simulink model "FX150_model"  (R2022a)
settings: Solver=ode4  StartTime=0.0  StopTime=35  FixedStep=0.001  RelTol=1e-3
PreLoadFcn:
  | filepath  = fileparts(get_param(bdroot, 'FileName'))
  | cd(filepath);
InitFcn:
  | Model_Params;
values from neighbouring files (symbols this model uses):
  aM = 0.03    [Model_Params.m]
  aT = 1.4874    [Model_Params.m]
  bT = -0.0147    [Model_Params.m]
  ModelParam_envAltitude = -50    [Model_Params.m]
  ModelParam_GlobalNoiseGainSwitch = 0.4    [Model_Params.m]
  ModelParam_GPSEphFinal = 0.3    [Model_Params.m]
  ModelParam_GPSEpvFinal = 0.4    [Model_Params.m]
  ModelParam_GPSFix3DFix = 3    [Model_Params.m]
  ModelParam_GPSSatsVisible = 10    [Model_Params.m]
  ModelParam_motorJm = 0    [Model_Params.m]
  ModelParam_noiseBaroCoupleWithSpeed = 0    [Model_Params.m]
  ModelParam_noiseGPSSampTime = 0.2    [Model_Params.m]
  ModelParam_noisePowerIMU = 0    [Model_Params.m]
  ModelParam_noisePowerOffGainAccel = 0.04    [Model_Params.m]
  ModelParam_noisePowerOffGainAccelZ = 0.03    [Model_Params.m]
  ModelParam_noisePowerOffGainGyro = 0.02    [Model_Params.m]
  ModelParam_noisePowerOffGainGyroZ = 0.025    [Model_Params.m]
  ModelParam_noisePowerOffGainMag = 0.02    [Model_Params.m]
  ModelParam_noisePowerOffGainMagZ = 0.035    [Model_Params.m]
  ModelParam_noisePowerOnGainAccel = 0.8    [Model_Params.m]
  ModelParam_noisePowerOnGainAccelZ = 4.5    [Model_Params.m]
  ModelParam_noisePowerOnGainGyro = 2    [Model_Params.m]
  ModelParam_noisePowerOnGainGyroZ = 1    [Model_Params.m]
  ModelParam_noisePowerOnGainMag = 0.025    [Model_Params.m]
  ModelParam_noisePowerOnGainMagZ = 0.05    [Model_Params.m]
  ModelParam_noiseSampleTimeAccel = 0.001    [Model_Params.m]
  ModelParam_noiseSampleTimeGyro = 0.001    [Model_Params.m]
  ModelParam_noiseSampleTimeMag = 0.01    [Model_Params.m]
  ModelParam_noiseUpperGPS = 0.5    [Model_Params.m]
  ModelParam_noiseUpperWindBodyRatio = 0    [Model_Params.m]
  ModelParam_noiseWindSampTime = 0.001    [Model_Params.m]
  ModelParam_timeSampBaro = 0.01    [Model_Params.m]
  ModelParam_uavCCm = [0.0123 0.0123 0.0121]    [Model_Params.m]
  ModelParam_uavCd = [0.6023, 0.6023, 0.9]    [Model_Params.m]
  ModelParam_uavMass = 0.3175    [Model_Params.m]
  ModelParam_uavR = 0.075    [Model_Params.m]
  ModelParam_uavType = int8(3)    [Model_Params.m]
  w1 = 0.3812e+04    (= 3812)    [Model_Params.m]
  w2 = -1.3923e+04    (= -13923)    [Model_Params.m]
  w3 = 3.1012e+04    (= 31012)    [Model_Params.m]
undefined symbols (not defined in the file or in its folder): Earth, ModelParam_GPSEpvInitial, ModelParam_GPSEpvTimeConstant, ModelParam_noiseLowPassFilterCoeAccel, ModelParam_noiseLowPassFilterCoeGyro, ModelParam_timeSamp, Newton, Raphson, WGS84
libraries: simulink x4, aerolibtransform2 x3, sharedtransform x3, aerolibasang x3, aerolibatmos2 x2, aerolibutil x2, aerolibconvert2 x1, aerolibobsolete x1, shared6dof x1, aerolibnav x1, aerolibgravity2 x1
(part 1 of 2)
settings Model: SimulationMode=accelerator  Creator=Jinrui  LastModifiedBy=Lenovo
settings SolverCC: AlgebraicLoopSolver=TrustRegion
settings DataIOCC: ReturnWorkspaceOutputs=off
settings OptimizationCC: ZeroExternalMemoryAtStartup=off  ZeroInternalMemoryAtStartup=off  EfficientTunableParamExpr=on
settings DebuggingCC: ParameterTunabilityLossMsg=error  UnconnectedInputMsg=warning  UnconnectedOutputMsg=warning  UnconnectedLineMsg=warning  SFMachineParentedDataDiag=warning  ArithmeticOperatorsInVariantConditions=warning
settings SFSimCC: SimUseLocalCustomCode=off  MATLABDynamicMemAlloc=off  CustomCodeUndefinedFunction=UseInterfaceOnly  SimTargetLang=C++
settings RTWCC: SystemTargetFile=ert.tlc  GenerateMakefile=off  PackageGeneratedCodeAndArtifacts=on  PackageName=MulticopterModel  TemplateMakefile=ert_default_tmf  RTWUseLocalCustomCode=off  TargetLang=C++  RTWCompilerOptimization=on
settings CodeAppCC: ForceParamTrailComments=on  OperatorAnnotations=on  SimulinkDataObjDesc=on  SFDataObjDesc=on  MATLABFcnDesc=on  InsertBlockDesc=on  StateflowObjectComments=on  MATLABSourceComments=on
settings ERTTargetCC: TargetLangStandard=C++03 (ISO)  MultiwordLength=2048  GenerateSampleERTMain=on  CodeInterfacePackaging=C++ class  SupportContinuousTime=on  MultiInstanceErrorCode=None  RootIOFormat=Structure reference  ERTCustomFileTemplate=example_file_process.tlc  ERTFilePackagingFormat=Compact
settings SimscapeCC: SimscapeNormalizeSystem=off

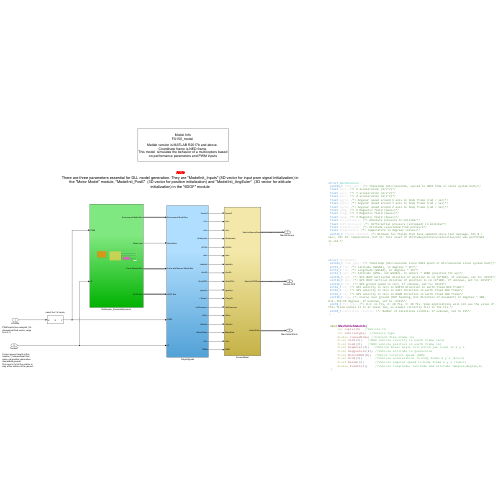
[thumbnail: Simulink's stored preview of the top-level diagram]
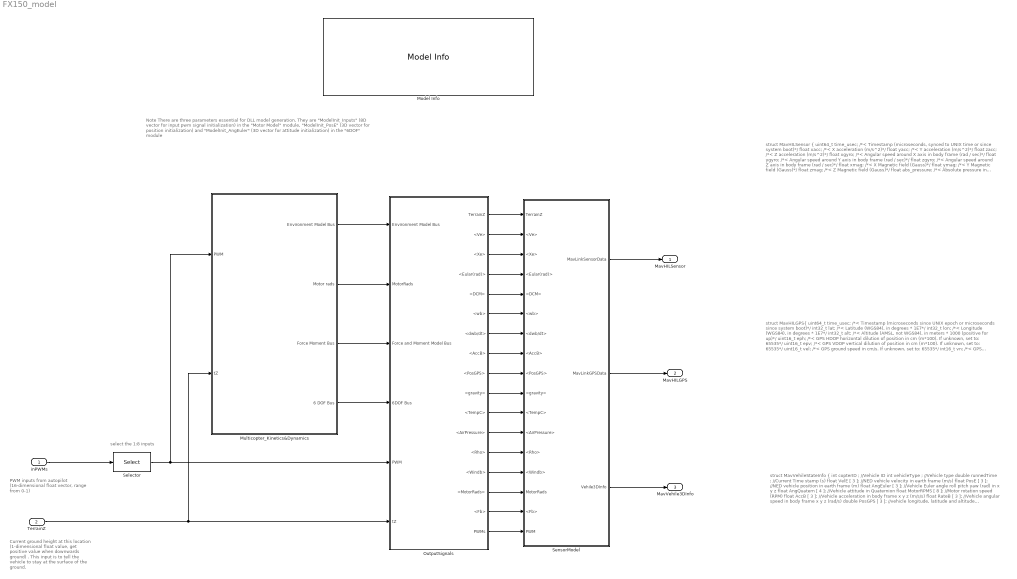
== system FX150_model ==
  note: PWM inputs from autopilot (16-dimensional float vector, range from 0-1)
  note: Note
      | There are three parameters essential for DLL model generation. They are "ModelInit_Inputs" (8D vector for input pwm signal initialization) in the "Motor Model" module, "ModelInit_PosE" (3D vector for position initialization) and "ModelInit_AngEuler" (3D vector for attitude initialization) in the "6DOF" module
  note: select the 1:8 inputs
  note: struct MavVehileStateInfo {
      | int copterID ; //Vehicle ID
      | int vehicleType ; //Vehicle type
      | double runnedTime ; //Current Time stamp (s)
      | float VelE [ 3 ]; //NED vehicle velocity in earth frame (m/s)
      | float PosE [ 3 ]; //NED vehicle position in earth frame (m)
      | float AngEuler [ 3 ]; //Vehicle Euler angle roll pitch yaw (rad) in x y z
      | float AngQuatern [ 4 ]; //Vehicle attitude in Quaternion
      | float MotorRPMS [ 8 ]; //Motor rotation speed (RPM)
      | float AccB [ 3 ]; //Vehicle acceleration in body frame x y z (m/s/s)
      | float RateB [ 3 ]; //Vehicle angular speed in body frame x y z (rad/s)
      | double PosGPS [ 3 ]; //vehicle longitude, latitude and altitude (degree,degree,m)
      | }
  note: struct MavHILGPS{
      | uint64_t time_usec; /*< Timestamp (microseconds since UNIX epoch or microseconds since system boot)*/
      | int32_t lat; /*< Latitude (WGS84), in degrees * 1E7*/
      | int32_t lon; /*< Longitude (WGS84), in degrees * 1E7*/
      | int32_t alt; /*< Altitude (AMSL, not WGS84), in meters * 1000 (positive for up)*/
      | uint16_t eph; /*< GPS HDOP horizontal dilution of position in cm (m*100). If unknown, set to: 65535*/
      | uint16_t epv; /*< GPS VDOP vertical dilution of position in cm (m*100). If unknown, set to: 65535*/
      | uint16_t vel; /*< GPS ground speed in cm/s. If unknown, set to: 65535*/
      | int16_t vn; /*< GPS velocity in cm/s in NORTH direction in earth-fixed NED frame*/
      | int16_t ve; /*< GPS velocity in cm/s in EAST direction in earth-fixed NED frame*/
      | int16_t vd; /*< GPS velocity in cm/s in DOWN direction in earth-fixed NED frame*/
      | uint16_t cog; /*< Course over ground (NOT heading, but direction of movement) in degrees * 100, 0.0..359.99 degrees. If unknown, set to: 65535*/
      | uint8_t fix_type; /*< 0-1: no fix, 2: 2D fix, 3: 3D fix. Some applications will not use the value of this field unless it is at least two, so always correctly fill in the fix.*/
      | uint8_t satellites_visible; /*< Number of satellites visible. If unknown, set to 255*/
      | }) ;
  note: struct MavHILSensor {
      | uint64_t time_usec; /*< Timestamp (microseconds, synced to UNIX time or since system boot)*/
      | float xacc; /*< X acceleration (m/s^2)*/
      | float yacc; /*< Y acceleration (m/s^2)*/
      | float zacc; /*< Z acceleration (m/s^2)*/
      | float xgyro; /*< Angular speed around X axis in body frame (rad / sec)*/
      | float ygyro; /*< Angular speed around Y axis in body frame (rad / sec)*/
      | float zgyro; /*< Angular speed around Z axis in body frame (rad / sec)*/
      | float xmag; /*< X Magnetic field (Gauss)*/
      | float ymag; /*< Y Magnetic field (Gauss)*/
      | float zmag; /*< Z Magnetic field (Gauss)*/
      | float abs_pressure; /*< Absolute pressure in millibar*/
      | float diff_pressure; /*< Differential pressure (airspeed) in millibar*/
      | float pressure_alt; /*< Altitude calculated from pressure*/
      | float temperature; /*< Temperature in degrees celsius*/
      | uint32_t fields_updated; /*< Bitmask for fields that have updated since last message, bit 0 = xacc, bit 12: temperature, bit 31: full reset of attitude/position/velocities/etc was performed in sim.*/
      | });
  note: Current ground height at this location (1-dimensional float value, get positive value when downwards ground) .
      | This input is to tell the vehicle to stay at the surface of the ground.
  inPWMs : Inport  PortDimensions=16
  TerrainZ : Inport  Port=2
  Model Info : simulink/Model-Wide Utilities/Model Info  Frame=on  DisplayStringWithTags=|  HorizontalTextAlignment=Center  LeftAlignmentValue=0.5
      | Model Info
      | %<ModelName> 
      | %<Description>   
      | Matlab version is MATLAB R2017b and above. 
      | Coordinate frame is NED frame.
      |  This model  simulates the behavior of a multicopters based 
      | on performance parameters and PWM inputs
  Multicopter_Kinetics&Dynamics : Subsystem
  OutputSignals : Subsystem
  Selector : Selector  InputPortWidth=16  IndexOptions=Index vector (dialog)  Indices=[1:8]  OutputSizes=1
  SensorModel : Subsystem
  MavHILSensor : Outport  OutDataTypeStr=Bus: MavLinkSensor  VectorParamsAs1DForOutWhenUnconnected=off
  MavHILGPS : Outport  Port=2  OutDataTypeStr=Bus: MavLinkGPS  VectorParamsAs1DForOutWhenUnconnected=off
  MavVehile3DInfo : Outport  Port=3  OutDataTypeStr=Bus: MavVehileInfo  VectorParamsAs1DForOutWhenUnconnected=off
  wires:
  inPWMs/1 -> Selector/1
  OutputSignals/9(<PosGPS>) -> SensorModel/9(<PosGPS>)
  SensorModel/2(MavLinkGPSData) -> MavHILGPS/1
  OutputSignals/1(TerrainZ) -> SensorModel/1(TerrainZ)
  OutputSignals/4(<Eular(rad)>) -> SensorModel/4(<Eular(rad)>)
  SensorModel/3(Vehile3DInfo) -> MavVehile3DInfo/1
  OutputSignals/2(<Ve>) -> SensorModel/2(<Ve>)
  OutputSignals/6(<wb>) -> SensorModel/6(<wb>)
  OutputSignals/5(<DCM>) -> SensorModel/5(<DCM>)
  SensorModel/1(MavLinkSensorData) -> MavHILSensor/1
  OutputSignals/15(<MotorRads>) -> SensorModel/15(MotorRads)
  OutputSignals/10(<gravity>) -> SensorModel/10(<gravity>)
  OutputSignals/7(<dwb/dt>) -> SensorModel/7(<dwb/dt>)
  OutputSignals/13(<Rho>) -> SensorModel/13(<Rho>)
  OutputSignals/3(<Xe>) -> SensorModel/3(<Xe>)
  OutputSignals/11(<TempC>) -> SensorModel/11(<TempC>)
  OutputSignals/12(<AirPressure>) -> SensorModel/12(<AirPressure>)
  OutputSignals/8(<AccB>) -> SensorModel/8(<AccB>)
  OutputSignals/16(<Fb>) -> SensorModel/16(<Fb>)
  OutputSignals/14(<Windb>) -> SensorModel/14(<Windb>)
  OutputSignals/17(PWMs) -> SensorModel/17(PWM)
  Selector/1 -> Multicopter_Kinetics&Dynamics/1(PWM), OutputSignals/5(PWM)
  Multicopter_Kinetics&Dynamics/1(Environment Model Bus) -> OutputSignals/1(Environment Model Bus)
  TerrainZ/1 -> Multicopter_Kinetics&Dynamics/2(tZ), OutputSignals/6(tZ)
  Multicopter_Kinetics&Dynamics/3(Force Moment Bus) -> OutputSignals/3(Force and Moment Model Bus)
  Multicopter_Kinetics&Dynamics/4(6 DOF Bus) -> OutputSignals/4(6DOF Bus)
  Multicopter_Kinetics&Dynamics/2(Motor rads) -> OutputSignals/2(MotorRads)

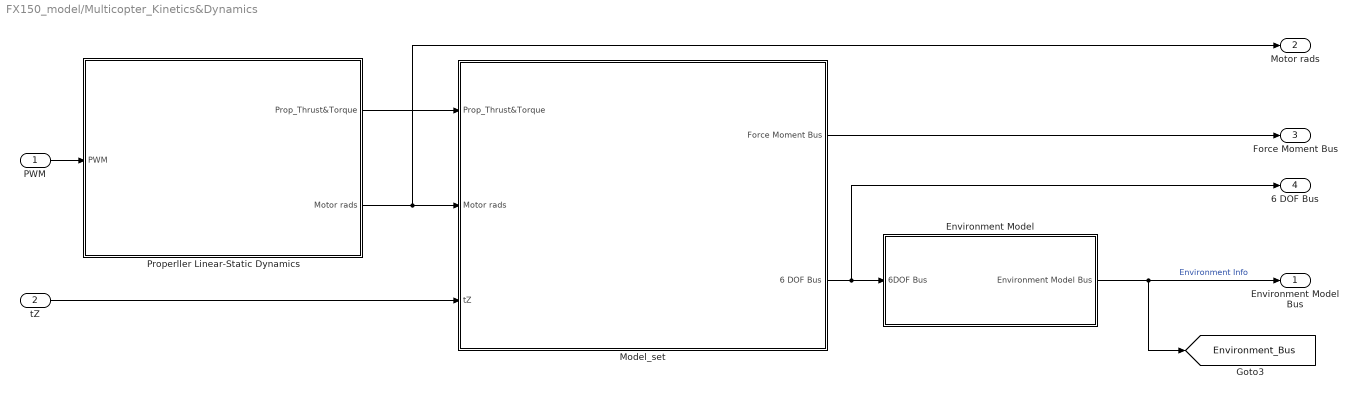
== system FX150_model/Multicopter_Kinetics&Dynamics ==
  PWM : Inport
  tZ : Inport  Port=2
  Environment Model : Subsystem
  Model_set : Subsystem
  Properller Linear-Static Dynamics : Subsystem  TreatAsAtomicUnit=on
  Environment Model Bus : Outport  VectorParamsAs1DForOutWhenUnconnected=off
  Motor rads : Outport  Port=2  VectorParamsAs1DForOutWhenUnconnected=off
  Force Moment Bus : Outport  Port=3  VectorParamsAs1DForOutWhenUnconnected=off
  6 DOF Bus : Outport  Port=4  VectorParamsAs1DForOutWhenUnconnected=off
  tag scope: Environment_Bus=global
  wires:
  Properller Linear-Static Dynamics/2(Motor rads) -> Motor rads/1, Model_set/2(Motor rads)
  tZ/1 -> Model_set/3(tZ)
  Model_set/2(6 DOF Bus) -> 6 DOF Bus/1, Environment Model/1(6DOF Bus)
  PWM/1 -> Properller Linear-Static Dynamics/1(PWM)
  Properller Linear-Static Dynamics/1(Prop_Thrust&Torque) -> Model_set/1(Prop_Thrust&Torque)
  Environment Model/1(Environment Model Bus) -> Environment Model Bus/1, [Environment_Bus]  "Environment Info"
  Model_set/1(Force Moment Bus) -> Force Moment Bus/1

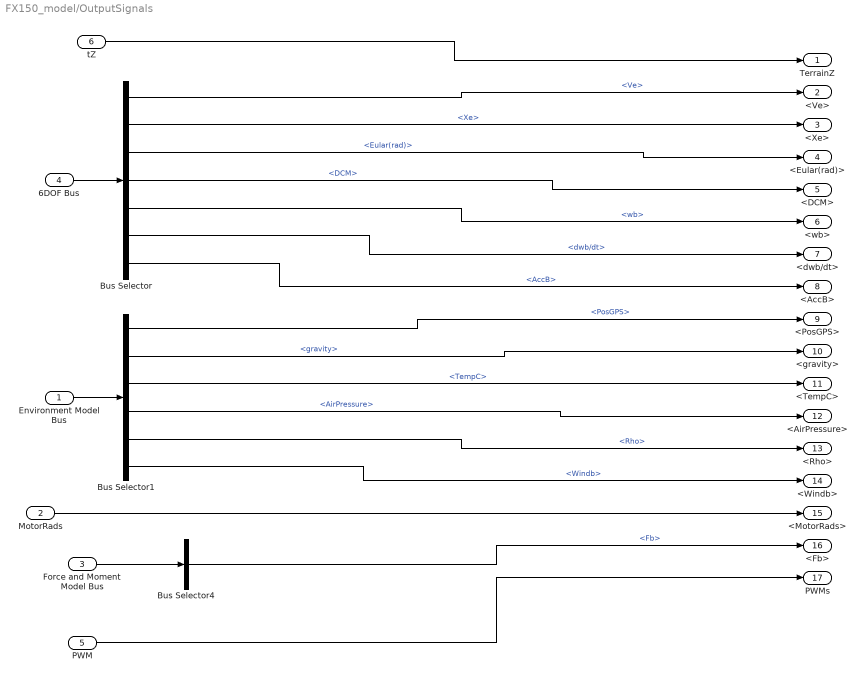
== system FX150_model/OutputSignals ==
  Environment Model Bus : Inport
  MotorRads : Inport  Port=2
  Force and Moment Model Bus : Inport  Port=3
  6DOF Bus : Inport  Port=4
  PWM : Inport  Port=5
  tZ : Inport  Port=6
  Bus Selector : BusSelector  OutputSignals=Ve,Xe,Eular(rad),DCM,wb,dwb/dt,AccB
  Bus Selector1 : BusSelector  OutputSignals=PosGPS,gravity,TempC,AirPressure,Rho,Windb
  Bus Selector4 : BusSelector  OutputSignals=Fb
  TerrainZ : Outport  VectorParamsAs1DForOutWhenUnconnected=off
  <Ve> : Outport  Port=2  VectorParamsAs1DForOutWhenUnconnected=off
  <Xe> : Outport  Port=3  VectorParamsAs1DForOutWhenUnconnected=off
  <Eular(rad)> : Outport  Port=4  VectorParamsAs1DForOutWhenUnconnected=off
  <DCM> : Outport  Port=5  VectorParamsAs1DForOutWhenUnconnected=off
  <wb> : Outport  Port=6  VectorParamsAs1DForOutWhenUnconnected=off
  <dwb/dt> : Outport  Port=7  VectorParamsAs1DForOutWhenUnconnected=off
  <AccB> : Outport  Port=8  VectorParamsAs1DForOutWhenUnconnected=off
  <PosGPS> : Outport  Port=9  VectorParamsAs1DForOutWhenUnconnected=off
  <gravity> : Outport  Port=10  VectorParamsAs1DForOutWhenUnconnected=off
  <TempC> : Outport  Port=11  VectorParamsAs1DForOutWhenUnconnected=off
  <AirPressure> : Outport  Port=12  VectorParamsAs1DForOutWhenUnconnected=off
  <Rho> : Outport  Port=13  VectorParamsAs1DForOutWhenUnconnected=off
  <Windb> : Outport  Port=14  VectorParamsAs1DForOutWhenUnconnected=off
  <MotorRads> : Outport  Port=15  VectorParamsAs1DForOutWhenUnconnected=off
  <Fb> : Outport  Port=16  VectorParamsAs1DForOutWhenUnconnected=off
  PWMs : Outport  Port=17  VectorParamsAs1DForOutWhenUnconnected=off
  wires:
  Force and Moment Model Bus/1 -> Bus Selector4/1
  MotorRads/1 -> <MotorRads>/1
  Bus Selector1/4 -> <AirPressure>/1  "<AirPressure>"
  Bus Selector/3 -> <Eular(rad)>/1  "<Eular(rad)>"
  Bus Selector1/6 -> <Windb>/1  "<Windb>"
  Bus Selector1/2 -> <gravity>/1  "<gravity>"
  PWM/1 -> PWMs/1
  Bus Selector/4 -> <DCM>/1  "<DCM>"
  Bus Selector/6 -> <dwb/dt>/1  "<dwb/dt>"
  Bus Selector1/1 -> <PosGPS>/1  "<PosGPS>"
  Bus Selector4/1 -> <Fb>/1  "<Fb>"
  Bus Selector/7 -> <AccB>/1  "<AccB>"
  Bus Selector/1 -> <Ve>/1  "<Ve>"
  Bus Selector/5 -> <wb>/1  "<wb>"
  Bus Selector/2 -> <Xe>/1  "<Xe>"
  Bus Selector1/5 -> <Rho>/1  "<Rho>"
  tZ/1 -> TerrainZ/1
  Bus Selector1/3 -> <TempC>/1  "<TempC>"
  Environment Model Bus/1 -> Bus Selector1/1
  6DOF Bus/1 -> Bus Selector/1

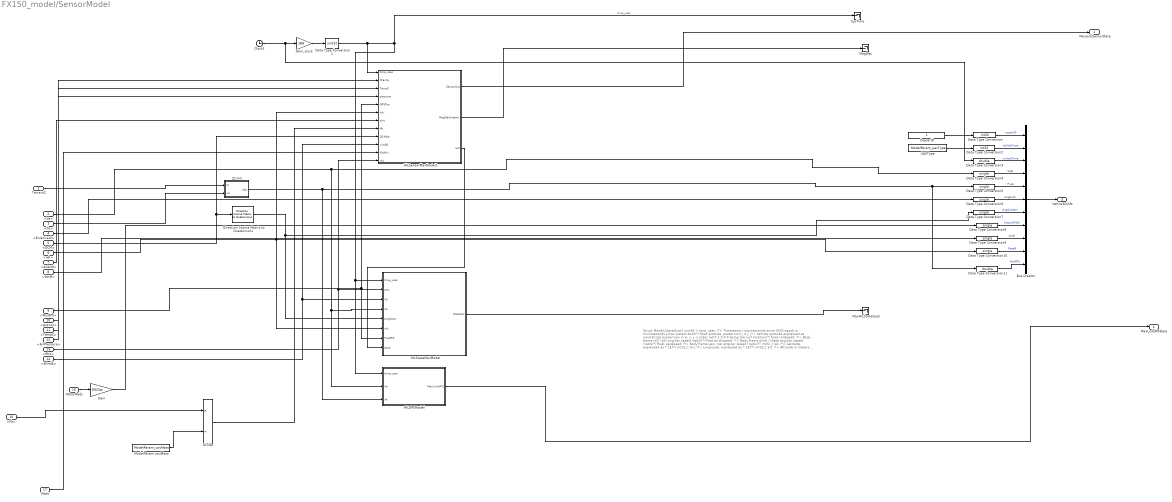
== system FX150_model/SensorModel ==
  note: Struct MavHILStateQuat{
      | uint64_t time_usec; /*< Timestamp (microseconds since UNIX epoch or microseconds since system boot)*/
      | float attitude_quaternion [ 4 ]; /*< Vehicle attitude expressed as normalized quaternion in w, x, y, z order (with 1 0 0 0 being the null-rotation)*/
      | float rollspeed; /*< Body frame roll / phi angular speed (rad/s)*/
      | float pitchspeed; /*< Body frame pitch / theta angular speed (rad/s)*/
      | float yawspeed; /*< Body frame yaw / psi angular speed (rad/s)*/
      | int32_t lat; /*< Latitude, expressed as * 1E7*/
      | int32_t lon; /*< Longitude, expressed as * 1E7*/
      | int32_t alt; /*< Altitude in meters, expressed as * 1000 (millimeters)*/
      | int16_t vx; /*< Ground X Speed (Latitude), expressed as cm/s*/
      | int16_t vy; /*< Ground Y Speed (Longitude), expressed as cm/s*/
      | int16_t vz; /*< Ground Z Speed (Altitude), expressed as cm/s*/
      | uint16_t ind_airspeed; /*< Indicated airspeed, expressed as cm/s*/
      | uint16_t true_airspeed; /*< True airspeed, expressed as cm/s*/
      | int16_t xacc; /*< X acceleration (mg)*/
      | int16_t yacc; /*< Y acceleration (mg)*/
      | int16_t zacc; /*< Z acceleration (mg)*/
      | };
  TerrainZ : Inport
  <Ve> : Inport  Port=2
  <Xe> : Inport  Port=3
  <Eular(rad)> : Inport  Port=4
  <DCM> : Inport  Port=5
  <wb> : Inport  Port=6
  <dwb/dt> : Inport  Port=7
  <AccB> : Inport  Port=8
  <PosGPS> : Inport  Port=9
  <gravity> : Inport  Port=10
  <TempC> : Inport  Port=11
  <AirPressure> : Inport  Port=12
  <Rho> : Inport  Port=13
  <Windb> : Inport  Port=14
  MotorRads : Inport  Port=15
  <Fb> : Inport  Port=16
  PWM : Inport  Port=17
  Bus Creator : BusCreator  Inputs=11  OutDataTypeStr=Bus: MavVehileInfo
  Clock1 : Clock
  CopterID : Constant
  Data Type Conversion : DataTypeConversion  OutDataTypeStr=int32  SaturateOnIntegerOverflow=off  RndMeth=Floor
  Data Type Conversion1 : DataTypeConversion  OutDataTypeStr=uint32  SaturateOnIntegerOverflow=off  RndMeth=Floor
  Data Type Conversion{4..10} (7 alike) : DataTypeConversion  OutDataTypeStr=single  SaturateOnIntegerOverflow=off  RndMeth=Floor
  Data Type Conversion11 : DataTypeConversion  OutDataTypeStr=double  SaturateOnIntegerOverflow=off  RndMeth=Floor
  Data Type Conversion2 : DataTypeConversion  OutDataTypeStr=int32  SaturateOnIntegerOverflow=off  RndMeth=Floor
  Data Type Conversion3 : DataTypeConversion  OutDataTypeStr=double  SaturateOnIntegerOverflow=off  RndMeth=Floor
  Direction Cosine Matrix to Quaternions : sharedtransform/Direction Cosine Matrix  to Quaternions  aMode=aMode  action=None  tolerance=eps(2)
      settings: SourceProductBaseCode=AE,PW,DR,MT,VE
  Divide : Product  Inputs=*/
  Gain : Gain  Gain=60/2/pi
  Gain_clock : Gain  Gain=1E6
  HILGPSModel : Subsystem
  HILSensorMavModel1 : Subsystem
  HILStateMavModel : Subsystem
  MagDec : Terminator
  MavHILStateQuat : Terminator
  ModelParam.uavMass : Constant  Value=ModelParam_uavMass
  SysTime : Terminator
  UAVType : Constant  Value=ModelParam_uavType
  ZLimit : MATLAB Function  TreatAsAtomicUnit=on
  MavLinkSensorData : Outport  VectorParamsAs1DForOutWhenUnconnected=off
  MavLinkGPSData : Outport  Port=2  VectorParamsAs1DForOutWhenUnconnected=off
  Vehile3DInfo : Outport  Port=3  VectorParamsAs1DForOutWhenUnconnected=off
  wires:
  <Xe>/1 -> ZLimit/2(xe)
  <PosGPS>/1 -> HILStateMavModel/7(PosGPS), HILSensorMavModel1/5(GPSPos)
  <TempC>/1 -> HILSensorMavModel1/3(TempC)
  <AirPressure>/1 -> HILSensorMavModel1/4(pressure)
  Clock1/1 -> Data Type Conversion3/1, Gain_clock/1
  Data Type Conversion1/1 -> HILSensorMavModel1/1(time_usec), SysTime/1, HILGPSModel/1(time_usec), HILStateMavModel/1(time_usec)  "time_usec"
  <gravity>/1 -> HILSensorMavModel1/2(Gravity)
  <Rho>/1 -> HILSensorMavModel1/12(rho), HILStateMavModel/2(pho)
  Gain_clock/1 -> Data Type Conversion1/1
  <DCM>/1 -> HILSensorMavModel1/9(DCMbe), Direction Cosine Matrix to Quaternions/1
  <Eular(rad)>/1 -> Data Type Conversion6/1
  <dwb/dt>/1 -> HILSensorMavModel1/7(dwt)
  <wb>/1 -> HILSensorMavModel1/6(wb), Data Type Conversion10/1, HILStateMavModel/6(wb)
  <Ve>/1 -> HILGPSModel/2(Ve), HILStateMavModel/4(Ve), Data Type Conversion4/1
  TerrainZ/1 -> ZLimit/1(zt)
  CopterID/1 -> Data Type Conversion/1
  HILSensorMavModel1/2(MagDeclination) -> MagDec/1
  <AccB>/1 -> Data Type Conversion9/1
  Divide/1 -> HILSensorMavModel1/8(Ab)
  Data Type Conversion5/1 -> Bus Creator/5  "PosE"
  Data Type Conversion7/1 -> Bus Creator/7  "AngQuatern"
  Data Type Conversion4/1 -> Bus Creator/4  "VelE"
  Data Type Conversion9/1 -> Bus Creator/9  "AccB"
  Data Type Conversion10/1 -> Bus Creator/10  "RateB"
  PWM/1 -> HILSensorMavModel1/11(PWMin)
  Data Type Conversion11/1 -> Bus Creator/11  "PosGPS"
  Data Type Conversion6/1 -> Bus Creator/6  "AngEuler"
  ZLimit/1(Xee) -> Data Type Conversion11/1, Data Type Conversion5/1, HILGPSModel/3(Xe)
  Data Type Conversion/1 -> Bus Creator/1  "copterID"
  Bus Creator/1 -> Vehile3DInfo/1
  <Fb>/1 -> Divide/1
  Gain/1 -> Data Type Conversion8/1
  HILStateMavModel/1(stateOut) -> MavHILStateQuat/1
  Data Type Conversion8/1 -> Bus Creator/8  "MotorRPMS"
  Direction Cosine Matrix to Quaternions/1 -> Data Type Conversion7/1, HILStateMavModel/5(AngQuat)
  UAVType/1 -> Data Type Conversion2/1
  Data Type Conversion3/1 -> Bus Creator/3  "runnedTime"
  HILSensorMavModel1/3(acc) -> HILStateMavModel/8(Accb)
  ModelParam.uavMass/1 -> Divide/2
  Data Type Conversion2/1 -> Bus Creator/2  "vehicleType"
  HILSensorMavModel1/1(SensorOut) -> MavLinkSensorData/1
  HILGPSModel/1(MavLinkGPS) -> MavLinkGPSData/1
  <Windb>/1 -> HILSensorMavModel1/10(windB), HILStateMavModel/3(Vb)
  MotorRads/1 -> Gain/1

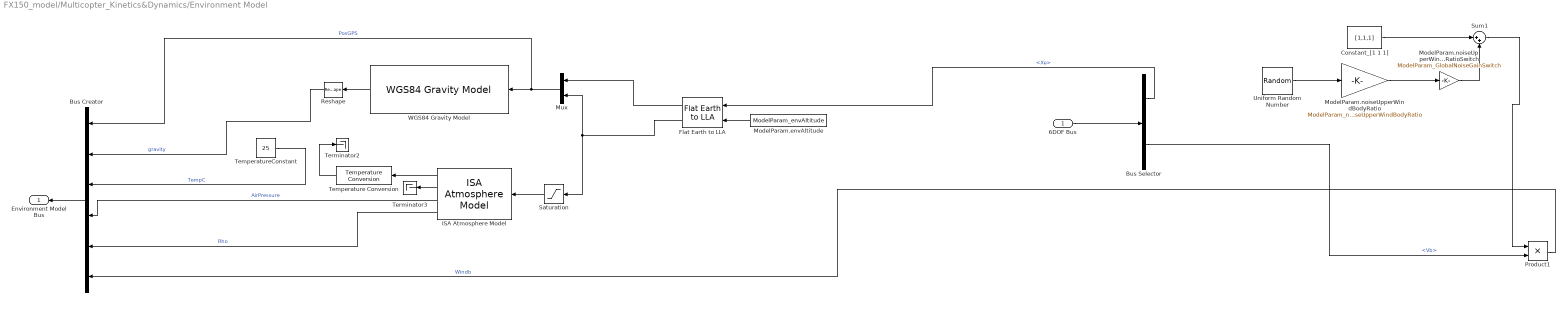
== system FX150_model/Multicopter_Kinetics&Dynamics/Environment Model ==
  6DOF Bus : Inport
  Bus Creator : BusCreator  Inputs=6
  Bus Selector : BusSelector  OutputSignals=Xe,Vb
  Constant_[1 1 1] : Constant  Value=[1,1,1]  VectorParams1D=off
  Flat Earth to LLA : aerolibtransform2/Flat Earth to LLA  units=Metric (MKS)  ptype=Earth (WGS84)  F=1/298.257223563  R=6378137  refPosPort=off  LL0=ModelParam_GPSLatLong  psi=0
  ISA Atmosphere Model : aerolibatmos2/ISA Atmosphere Model  custom=off  g=9.80665  gamma=1.4  R=287.0531  L=0.0065  h_trop=11000  h_strat=20000  rho0=1.225  P0=101325  T0=288.15  h0=0
  ModelParam.envAltitude : Constant  Value=ModelParam_envAltitude
  ModelParam.noiseUpperWindBodyRatio : Gain  Gain=ModelParam_noiseUpperWindBodyRatio
  ModelParam.noiseUpperWindBodyRatioSwitch : Gain  Gain=ModelParam_GlobalNoiseGainSwitch
  Mux : Mux  Inputs=2
  Product1 : Product
  Reshape : Reshape
  Saturation : Saturate  UpperLimit=100000  LowerLimit=0
  Sum1 : Sum  Inputs=|++
  Temperature Conversion : aerolibconvert2/Temperature Conversion  IU=K  OU=C
      settings: SourceProductBaseCode=AE
  TemperatureConstant : Constant  Value=25
  Terminator2 : Terminator
  Terminator3 : Terminator
  Uniform Random Number : UniformRandomNumber  Minimum=[-1,-1,-0.5]  Maximum=[1,1,0.5]  Seed=[564565,6846798,46545]  SampleTime=ModelParam_noiseWindSampTime
  "WGS84 Gravity Model " : aerolibobsolete/WGS84 Gravity Model   model=WGS84 Taylor Series  units=Metric (MKS)  no_atmos=on  precessing=on  jd_loc=off  month=October  day=10  year=2004  no_centrifugal=on  action=Warning
      settings: SourceProductBaseCode=AE
  Environment Model Bus : Outport  VectorParamsAs1DForOutWhenUnconnected=off
  wires:
  "WGS84 Gravity Model "/1 -> Reshape/1
  Reshape/1 -> Bus Creator/2  "gravity"
  ISA Atmosphere Model/1 -> Temperature Conversion/1
  ISA Atmosphere Model/2 -> Terminator3/1
  ISA Atmosphere Model/3 -> Bus Creator/4  "AirPressure"
  ISA Atmosphere Model/4 -> Bus Creator/5  "Rho"
  ModelParam.envAltitude/1 -> Flat Earth to LLA/2
  Mux/1 -> Bus Creator/1, "WGS84 Gravity Model "/1  "PosGPS"
  Flat Earth to LLA/1 -> Mux/1
  Bus Selector/2 -> Product1/2  "<Vb>"
  Uniform Random Number/1 -> ModelParam.noiseUpperWindBodyRatio/1
  Product1/1 -> Bus Creator/6  "Windb"
  Constant_[1 1 1]/1 -> Sum1/1
  ModelParam.noiseUpperWindBodyRatio/1 -> ModelParam.noiseUpperWindBodyRatioSwitch/1
  Sum1/1 -> Product1/1
  Temperature Conversion/1 -> Terminator2/1
  TemperatureConstant/1 -> Bus Creator/3  "TempC"
  ModelParam.noiseUpperWindBodyRatioSwitch/1 -> Sum1/2
  6DOF Bus/1 -> Bus Selector/1
  Bus Selector/1 -> Flat Earth to LLA/1  "<Xe>"
  Bus Creator/1 -> Environment Model Bus/1
  Flat Earth to LLA/2 -> Mux/2, Saturation/1
  Saturation/1 -> ISA Atmosphere Model/1

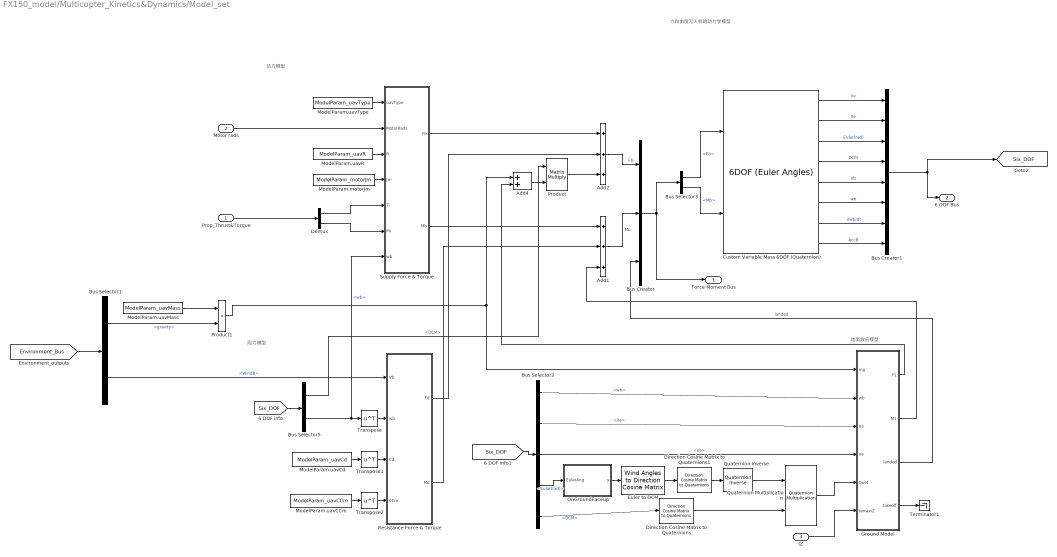
== system FX150_model/Multicopter_Kinetics&Dynamics/Model_set ==
  note: 地面效应模型
  note: 六自由度无人机的动力学模型
  note: 阻力模型
  note: 动力模型
  Prop_Thrust&Torque : Inport
  Motor rads : Inport  Port=2
  tZ : Inport  Port=3
  Add1 : Sum  Inputs=+++
  Add2 : Sum  Inputs=+++
  Add4 : Sum
  Bus Creator : BusCreator  Inputs=3
  Bus Creator1 : BusCreator  Inputs=8
  Bus Selector1 : BusSelector  OutputSignals=gravity,Windb
  Bus Selector2 : BusSelector  OutputSignals=wb,Xe,Ve,Eular(rad),DCM
  Bus Selector3 : BusSelector  OutputSignals=Fb,Mb
  Bus Selector5 : BusSelector  OutputSignals=DCM,wb
  Custom Variable Mass 6DOF (Quaternion) : shared6dof/6DOF (Euler Angles)  units=Metric (MKS)  mtype=Fixed  rep=Quaternion  xme_0=ModelInit_PosE  Vm_0=ModelInit_VelB  eul_0=ModelInit_AngEuler  pm_0=ModelInit_RateB  mass_0=ModelParam_uavMass  mass_e=0.5  mass_f=2.0  inertia=ModelParam_uavJ  inertia_e=eye(3)  inertia_f=2*eye(3)  k_quat=1.0  vre_flag=off  abi_flag=off  aMode=aMode  xme_statename=''  Vm_statename=''  eul_statename=''  quat_statename=''  pm_statename=''  mass_statename=''
      settings: SourceProductBaseCode=AE,PW,DR,MT,VE
  Demux : Demux  Outputs=2
  Direction Cosine Matrix to Quaternions : sharedtransform/Direction Cosine Matrix  to Quaternions  aMode=aMode  action=None  tolerance=eps(2)
      settings: SourceProductBaseCode=AE,PW,DR,MT,VE
  Direction Cosine Matrix to Quaternions1 : sharedtransform/Direction Cosine Matrix  to Quaternions  aMode=aMode  action=None  tolerance=eps(2)
      settings: SourceProductBaseCode=AE,PW,DR,MT,VE
  Euler to DCM : aerolibtransform2/Wind Angles to  Direction Cosine Matrix
      settings: SourceProductBaseCode=AE
  Ground Model : MATLAB Function  TreatAsAtomicUnit=on
  ModelParam.motorJm : Constant  Value=ModelParam_motorJm
  ModelParam.uavCCm : Constant  Value=ModelParam_uavCCm
  ModelParam.uavCd : Constant  Value=ModelParam_uavCd
  ModelParam.uavMass : Constant  Value=ModelParam_uavMass
  ModelParam.uavR : Constant  Value=ModelParam_uavR
  ModelParam.uavType : Constant  Value=ModelParam_uavType
  OnGroundFaceup : MATLAB Function  TreatAsAtomicUnit=on
  Product : Product  Multiplication=Matrix(*)
  Product1 : Product
  Quaternion Inverse : aerolibutil/Quaternion Inverse
  Quaternion Multiplication : aerolibutil/Quaternion Multiplication
  Resistance Force & Torque : MATLAB Function  TreatAsAtomicUnit=on
  Supply Force & Torque : MATLAB Function  TreatAsAtomicUnit=on
  Terminator1 : Terminator
  Transpose : Math  Operator=transpose  SignedPower=on
  Transpose1 : Math  Operator=transpose  SignedPower=on
  Transpose2 : Math  Operator=transpose  SignedPower=on
  Force Moment Bus : Outport  VectorParamsAs1DForOutWhenUnconnected=off
  6 DOF Bus : Outport  Port=2  VectorParamsAs1DForOutWhenUnconnected=off
  tag scope: Six_DOF=global
  wires:
  Bus Selector5/1 -> Product/1  "<DCM>"
  ModelParam.uavMass/1 -> Product1/1
  Transpose/1 -> Resistance Force & Torque/2(wb)
  Product1/1 -> Add4/1, Ground Model/1(mg)
  ModelParam.uavCd/1 -> Transpose1/1
  Supply Force & Torque/1(Fb) -> Add2/1
  Bus Selector2/4 -> OnGroundFaceup/1(EulerAng)  "<Eular(rad)>"
  Direction Cosine Matrix to Quaternions/1 -> Quaternion Multiplication/2
  ModelParam.uavR/1 -> Supply Force & Torque/3(R)
  Resistance Force & Torque/1(Fd) -> Add2/2
  Resistance Force & Torque/2(Md) -> Add1/2
  ModelParam.uavCCm/1 -> Transpose2/1
  Quaternion Inverse/1 -> Quaternion Multiplication/1
  ModelParam.motorJm/1 -> Supply Force & Torque/4(Jm)
  ModelParam.uavType/1 -> Supply Force & Torque/1(uavType)
  Bus Selector5/2 -> Supply Force & Torque/7(wb), Transpose/1  "<wb>"
  Demux/2 -> Supply Force & Torque/6(Mi)
  Transpose2/1 -> Resistance Force & Torque/4(CCm)
  Add1/1 -> Bus Creator/2  "Mb"
  Bus Selector2/3 -> Ground Model/4(Ve)  "<Ve>"
  Prop_Thrust&Torque/1 -> Demux/1
  [Six_DOF] -> Bus Selector5/1
  Product/1 -> Add2/3
  Demux/1 -> Supply Force & Torque/5(Ti)
  Bus Selector1/1 -> Product1/2  "<gravity>"
  Motor rads/1 -> Supply Force & Torque/2(MotorRads)
  Supply Force & Torque/2(Mb) -> Add1/1
  Bus Selector1/2 -> Resistance Force & Torque/1(Vb)  "<Windb>"
  Add2/1 -> Bus Creator/1  "Fb"
  [Six_DOF] -> Bus Selector2/1
  [Environment_Bus] -> Bus Selector1/1
  Transpose1/1 -> Resistance Force & Torque/3(Cd)
  Ground Model/4(takeoff) -> Terminator1/1
  Bus Selector2/5 -> Direction Cosine Matrix to Quaternions/1  "<DCM>"
  Quaternion Multiplication/1 -> Ground Model/5(Quet)
  tZ/1 -> Ground Model/6(terrainZ)
  Add4/1 -> Product/2
  Ground Model/3(landed) -> Bus Creator/3  "landed"
  Bus Selector2/1 -> Ground Model/2(wb)  "<wb>"
  Bus Selector2/2 -> Ground Model/3(Xe)  "<Xe>"
  Direction Cosine Matrix to Quaternions1/1 -> Quaternion Inverse/1
  OnGroundFaceup/1(y) -> Euler to DCM/1
  Euler to DCM/1 -> Direction Cosine Matrix to Quaternions1/1
  Ground Model/1(F1) -> Add4/2
  Ground Model/2(M1) -> Add1/3
  Bus Selector3/1 -> Custom Variable Mass 6DOF (Quaternion)/1  "<Fb>"
  Custom Variable Mass 6DOF (Quaternion)/7 -> Bus Creator1/7  "dwb/dt"
  Bus Creator/1 -> Bus Selector3/1, Force Moment Bus/1
  Custom Variable Mass 6DOF (Quaternion)/1 -> Bus Creator1/1  "Ve"
  Custom Variable Mass 6DOF (Quaternion)/2 -> Bus Creator1/2  "Xe"
  Bus Creator1/1 -> 6 DOF Bus/1, [Six_DOF]
  Custom Variable Mass 6DOF (Quaternion)/8 -> Bus Creator1/8  "AccB"
  Custom Variable Mass 6DOF (Quaternion)/6 -> Bus Creator1/6  "wb"
  Custom Variable Mass 6DOF (Quaternion)/5 -> Bus Creator1/5  "Vb"
  Bus Selector3/2 -> Custom Variable Mass 6DOF (Quaternion)/2  "<Mb>"
  Custom Variable Mass 6DOF (Quaternion)/4 -> Bus Creator1/4  "DCM"
  Custom Variable Mass 6DOF (Quaternion)/3 -> Bus Creator1/3  "Eular(rad)"

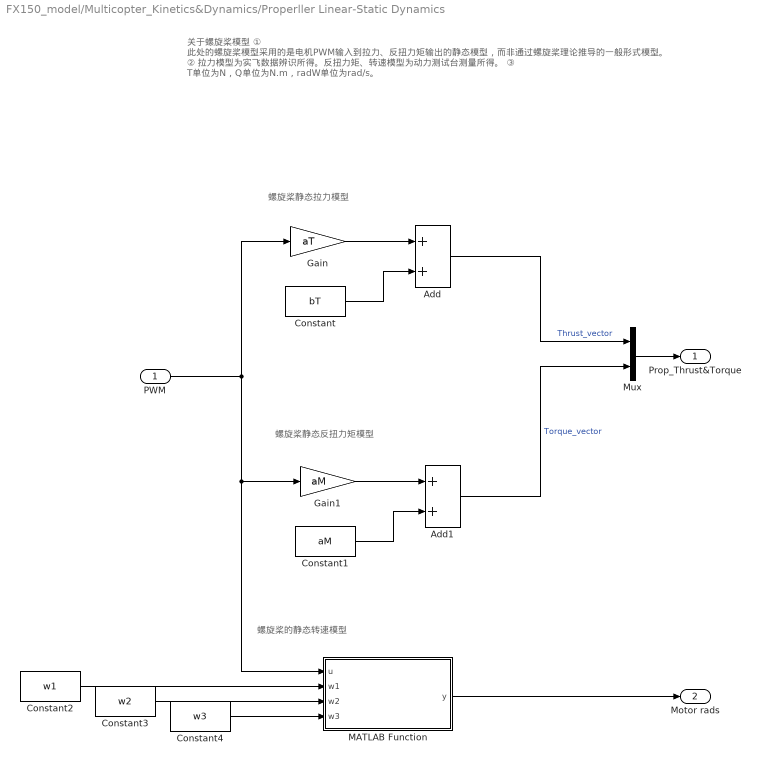
== system FX150_model/Multicopter_Kinetics&Dynamics/Properller Linear-Static Dynamics ==
  note: 螺旋桨的静态转速模型
  note: 关于螺旋桨模型
      | ① 此处的螺旋桨模型采用的是电机PWM输入到拉力、反扭力矩输出的静态模型，而非通过螺旋桨理论推导的一般形式模型。
      | ② 拉力模型为实飞数据辨识所得。反扭力矩、转速模型为动力测试台测量所得。
      | ③ T单位为N，Q单位为N.m，radW单位为rad/s。
  note: 螺旋桨静态反扭力矩模型
  note: 螺旋桨静态拉力模型
  PWM : Inport
  Add : Sum
  Add1 : Sum
  Constant : Constant  Value=bT
  Constant1 : Constant  Value=aM
  Constant2 : Constant  Value=w1
  Constant3 : Constant  Value=w2
  Constant4 : Constant  Value=w3
  Gain : Gain  Gain=aT
  Gain1 : Gain  Gain=aM
  MATLAB Function : MATLAB Function  TreatAsAtomicUnit=on
  Mux : Mux  Inputs=2
  Prop_Thrust&Torque : Outport  VectorParamsAs1DForOutWhenUnconnected=off
  Motor rads : Outport  Port=2  VectorParamsAs1DForOutWhenUnconnected=off
  wires:
  Gain/1 -> Add/1
  Constant/1 -> Add/2
  Add/1 -> Mux/1  "Thrust_vector"
  Add1/1 -> Mux/2  "Torque_vector"
  Constant1/1 -> Add1/2
  Gain1/1 -> Add1/1
  Mux/1 -> Prop_Thrust&Torque/1
  MATLAB Function/1(y) -> Motor rads/1
  PWM/1 -> Gain/1, MATLAB Function/1(u), Gain1/1
  Constant2/1 -> MATLAB Function/2(w1)
  Constant3/1 -> MATLAB Function/3(w2)
  Constant4/1 -> MATLAB Function/4(w3)

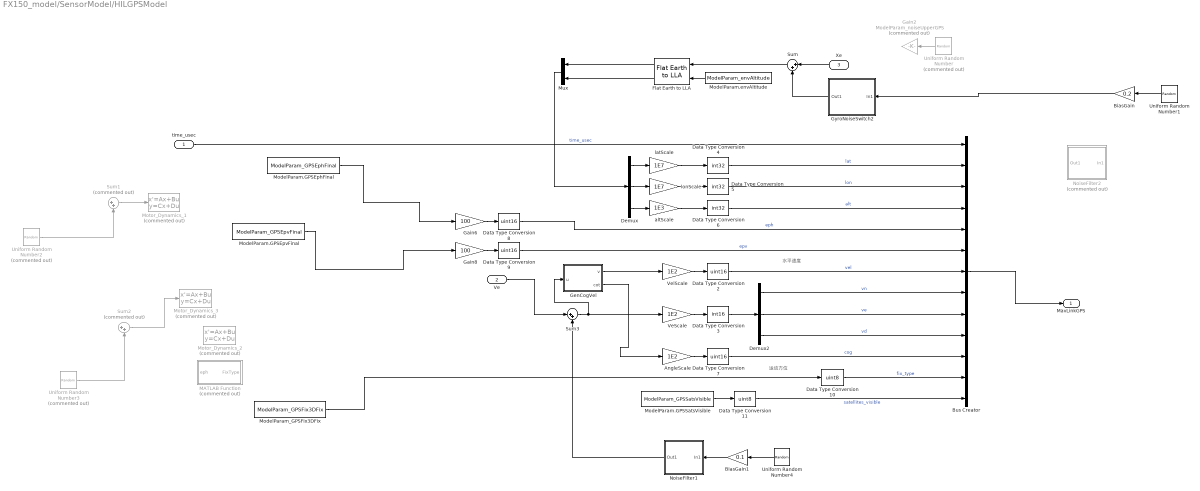
== system FX150_model/SensorModel/HILGPSModel ==
  note: 水平速度
  note: 运动方位
  time_usec : Inport
  Ve : Inport  Port=2
  Xe : Inport  Port=3
  AngleScale : Gain  Gain=1E2
  BiasGain : Gain  Gain=0.2
  BiasGain1 : Gain  Gain=0.1
  Bus Creator : BusCreator  Inputs=13  OutDataTypeStr=Bus: MavLinkGPS  NonVirtualBus=on
  Data Type Conversion10 : DataTypeConversion  OutDataTypeStr=uint8  RndMeth=Round  SaturateOnIntegerOverflow=off
  Data Type Conversion11 : DataTypeConversion  OutDataTypeStr=uint8  RndMeth=Round  SaturateOnIntegerOverflow=off
  Data Type Conversion{2,7..9} (4 alike) : DataTypeConversion  OutDataTypeStr=uint16  RndMeth=Round  SaturateOnIntegerOverflow=off
  Data Type Conversion3 : DataTypeConversion  OutDataTypeStr=int16  RndMeth=Round  SaturateOnIntegerOverflow=off
  Data Type Conversion4 : DataTypeConversion  OutDataTypeStr=int32  RndMeth=Round  SaturateOnIntegerOverflow=off
  Data Type Conversion5 : DataTypeConversion  OutDataTypeStr=int32  RndMeth=Round  SaturateOnIntegerOverflow=off
  Data Type Conversion6 : DataTypeConversion  OutDataTypeStr=int32  RndMeth=Round  SaturateOnIntegerOverflow=off
  Demux : Demux  Outputs=3
  Demux2 : Demux  Outputs=3
  Flat Earth to LLA : aerolibtransform2/Flat Earth to LLA  units=Metric (MKS)  ptype=Earth (WGS84)  F=1/298.257223563  R=6378137  refPosPort=off  LL0=ModelParam_GPSLatLong  psi=0
  Gain2 : Gain  Commented=on  Gain=ModelParam_noiseUpperGPS
  Gain6 : Gain  Gain=100
  Gain8 : Gain  Gain=100
  GenCogVel : MATLAB Function  TreatAsAtomicUnit=on
  GyroNoiseSwitch2 : Subsystem
  MATLAB Function : MATLAB Function  Commented=on  TreatAsAtomicUnit=on
  ModelParam.GPSEphFinal : Constant  Value=ModelParam_GPSEphFinal
  ModelParam.GPSEpvFinal : Constant  Value=ModelParam_GPSEpvFinal
  ModelParam.GPSSatsVisible : Constant  Value=ModelParam_GPSSatsVisible
  ModelParam.envAltitude : Constant  Value=ModelParam_envAltitude
  ModelParam_GPSFix3DFix : Constant  Value=ModelParam_GPSFix3DFix
  Motor_Dynamics_1 : StateSpace  Commented=on  A=-1/0.2  C=1/0.2  D=0  InitialCondition=20*0.2
  Motor_Dynamics_2 : StateSpace  Commented=on  A=-1/ModelParam_GPSEpvTimeConstant  C=1/ModelParam_GPSEpvTimeConstant  D=0  InitialCondition=ModelParam_GPSEpvInitial*ModelParam_GPSEpvTimeConstant
  Motor_Dynamics_3 : StateSpace  Commented=on  A=-1/0.2  C=1/0.2  D=0  InitialCondition=20*0.2
  Mux : Mux  Inputs=2
  NoiseFilter1 : Subsystem
  NoiseFilter2 : Subsystem  Commented=on
  Sum : Sum  Inputs=|++
  Sum1 : Sum  Commented=on  Inputs=|++
  Sum2 : Sum  Commented=on  Inputs=|++
  Sum3 : Sum  Inputs=|++
  Uniform Random Number : UniformRandomNumber  Commented=on  Minimum=[-1,-1,-3]  Maximum=[1,1,3]  Seed=[14524,7875,698]  SampleTime=ModelParam_timeSamp
  Uniform Random Number1 : UniformRandomNumber  Minimum=[-1,-1,-2]  Maximum=[1,1,2]  Seed=[1452,787,69]  SampleTime=ModelParam_noiseGPSSampTime
  Uniform Random Number2 : UniformRandomNumber  Commented=on  Minimum=-0.01  Maximum=0.01  Seed=4345454  SampleTime=ModelParam_noiseGPSSampTime
  Uniform Random Number3 : UniformRandomNumber  Commented=on  Seed=3244333  SampleTime=ModelParam_noiseGPSSampTime
  Uniform Random Number4 : UniformRandomNumber  Minimum=[-1,-1,-2]  Maximum=[1,1,2]  Seed=[5445,45433,33433]  SampleTime=ModelParam_noiseGPSSampTime
  VeScale : Gain  Gain=1E2
  VelScale : Gain  Gain=1E2
  altScale : Gain  Gain=1E3
  latScale : Gain  Gain=1E7
  lonScale : Gain  Gain=1E7
  MavLinkGPS : Outport  VectorParamsAs1DForOutWhenUnconnected=off
  wires:
  Data Type Conversion8/1 -> Bus Creator/5  "eph"
  Gain8/1 -> Data Type Conversion9/1
  Gain6/1 -> Data Type Conversion8/1
  Data Type Conversion9/1 -> Bus Creator/6  "epv"
  time_usec/1 -> Bus Creator/1  "time_usec"
  latScale/1 -> Data Type Conversion4/1
  lonScale/1 -> Data Type Conversion5/1
  altScale/1 -> Data Type Conversion6/1
  Data Type Conversion4/1 -> Bus Creator/2  "lat"
  Data Type Conversion5/1 -> Bus Creator/3  "lon"
  Data Type Conversion6/1 -> Bus Creator/4  "alt"
  Demux2/1 -> Bus Creator/8  "vn"
  Demux2/2 -> Bus Creator/9  "ve"
  Demux2/3 -> Bus Creator/10  "vd"
  VeScale/1 -> Data Type Conversion3/1
  Data Type Conversion3/1 -> Demux2/1
  VelScale/1 -> Data Type Conversion2/1
  Data Type Conversion2/1 -> Bus Creator/7  "vel"
  AngleScale/1 -> Data Type Conversion7/1
  Data Type Conversion7/1 -> Bus Creator/11  "cog"
  Data Type Conversion11/1 -> Bus Creator/13  "satellites_visible"
  Data Type Conversion10/1 -> Bus Creator/12  "fix_type"
  ModelParam.GPSSatsVisible/1 -> Data Type Conversion11/1
  Flat Earth to LLA/2 -> Mux/2
  ModelParam.envAltitude/1 -> Flat Earth to LLA/2
  Xe/1 -> Sum/1
  Flat Earth to LLA/1 -> Mux/1
  Demux/1 -> latScale/1
  Demux/2 -> lonScale/1
  Demux/3 -> altScale/1
  Uniform Random Number/1 -> Gain2/1
  Sum/1 -> Flat Earth to LLA/1
  Uniform Random Number1/1 -> BiasGain/1
  BiasGain/1 -> GyroNoiseSwitch2/1(In1)
  Mux/1 -> Demux/1
  ModelParam.GPSEphFinal/1 -> Gain6/1
  Sum2/1 -> Motor_Dynamics_3/1
  ModelParam_GPSFix3DFix/1 -> Data Type Conversion10/1
  Ve/1 -> Sum3/1
  GenCogVel/1(v) -> VelScale/1
  GyroNoiseSwitch2/1(Out1) -> Sum/2
  Bus Creator/1 -> MavLinkGPS/1
  BiasGain1/1 -> NoiseFilter1/1(In1)
  Uniform Random Number4/1 -> BiasGain1/1
  GenCogVel/2(cot) -> AngleScale/1
  Sum1/1 -> Motor_Dynamics_1/1
  Uniform Random Number2/1 -> Sum1/2
  Uniform Random Number3/1 -> Sum2/2
  ModelParam.GPSEpvFinal/1 -> Gain8/1
  Sum3/1 -> GenCogVel/1(u), VeScale/1
  NoiseFilter1/1(Out1) -> Sum3/2

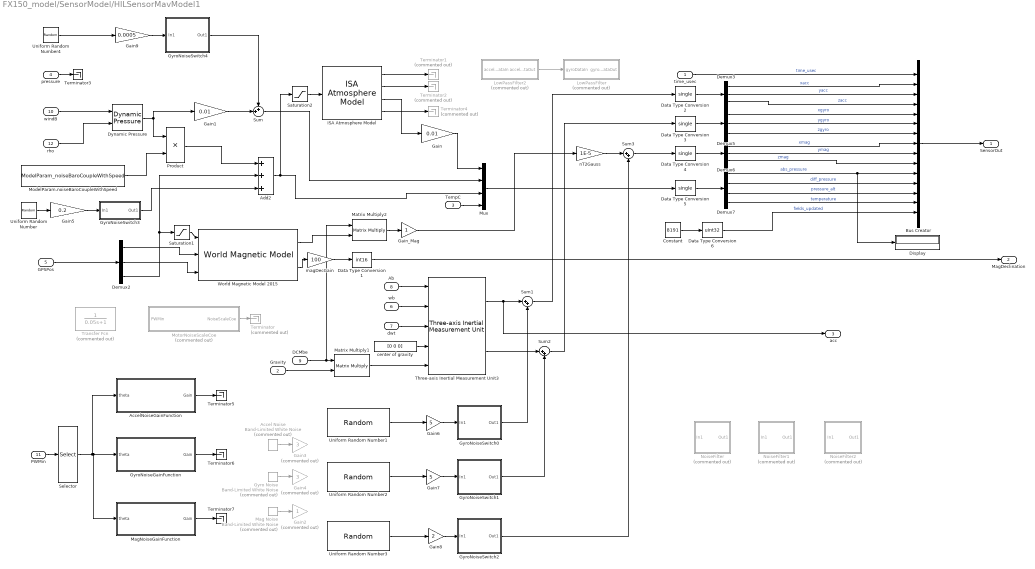
== system FX150_model/SensorModel/HILSensorMavModel1 ==
  time_usec : Inport
  Gravity : Inport  Port=2
  TempC : Inport  Port=3
  pressure : Inport  Port=4
  GPSPos : Inport  Port=5
  wb : Inport  Port=6
  dwt : Inport  Port=7
  Ab : Inport  Port=8
  DCMbe : Inport  Port=9
  windB : Inport  Port=10
  PWMin : Inport  Port=11
  rho : Inport  Port=12
  Accel Noise : simulink/Sources/Band-Limited White Noise  Commented=on  Cov=ModelParam_noisePowerAccel  Ts=ModelParam_noiseSampleTimeAccel  seed=[411144,1416,71144]
  AccelNoiseGainFunction : MATLAB Function  TreatAsAtomicUnit=on
  Add2 : Sum  Inputs=+++
  Bus Creator : BusCreator  Inputs=15  OutDataTypeStr=Bus: MavLinkSensor  NonVirtualBus=on
  Constant : Constant  Value=8191
  Data Type Conversion1 : DataTypeConversion  OutDataTypeStr=int16  SaturateOnIntegerOverflow=off  RndMeth=Floor
  Data Type Conversion{2..5} (4 alike) : DataTypeConversion  OutDataTypeStr=single  SaturateOnIntegerOverflow=off  RndMeth=Floor
  Data Type Conversion6 : DataTypeConversion  OutDataTypeStr=uint32  SaturateOnIntegerOverflow=off  RndMeth=Floor
  Demux{2..3,5..6} (4 alike) : Demux  Outputs=3
  Demux7 : Demux
  Display : Display
  Dynamic Pressure : aerolibasang/Dynamic Pressure
  Gain : Gain  Gain=0.01
  Gain1 : Gain  Gain=0.01
  Gain2 : Gain  Commented=on
  Gain3 : Gain  Commented=on  Gain=3
  Gain4 : Gain  Commented=on  Gain=3
  Gain5 : Gain  Gain=0.2
  Gain6 : Gain  Gain=5
  Gain7 : Gain  Gain=5
  Gain8 : Gain  Gain=2
  Gain9 : Gain  Gain=0.0005
  Gain_Mag : Gain
  Gyro Noise : simulink/Sources/Band-Limited White Noise  Commented=on  Cov=ModelParam_noisePowerGyro  Ts=ModelParam_noiseSampleTimeGyro  seed=[111,116,144]
  GyroNoiseGainFunction : MATLAB Function  TreatAsAtomicUnit=on
  GyroNoiseSwitch0 : Subsystem
  GyroNoiseSwitch1 : Subsystem
  GyroNoiseSwitch2 : Subsystem
  GyroNoiseSwitch3 : Subsystem
  GyroNoiseSwitch4 : Subsystem
  ISA Atmosphere Model : aerolibatmos2/ISA Atmosphere Model  custom=off  g=9.80665  gamma=1.4  R=287.0531  L=0.0065  h_trop=11000  h_strat=20000  rho0=1.225  P0=101325  T0=288.15  h0=0
  LowPassFilter : Subsystem  Commented=on
  LowPassFilter2 : Subsystem  Commented=on
  Mag Noise : simulink/Sources/Band-Limited White Noise  Commented=on  Cov=ModelParam_noisePowerMag  Ts=ModelParam_noiseSampleTimeMag  seed=[114,11699,999144]
  MagNoiseGainFunction : MATLAB Function  TreatAsAtomicUnit=on
  Matrix Multiply1 : Product  Multiplication=Matrix(*)
  Matrix Multiply2 : Product  Multiplication=Matrix(*)
  ModelParam.noiseBaroCoupleWithSpeed : Constant  Value=ModelParam_noiseBaroCoupleWithSpeed
  MotorNoiseScaleCoe : MATLAB Function  Commented=on  TreatAsAtomicUnit=on
  Mux : Mux
  NoiseFilter : Subsystem  Commented=on
  NoiseFilter1 : Subsystem  Commented=on
  NoiseFilter2 : Subsystem  Commented=on
  Product : Product
  Saturation1 : Saturate  UpperLimit=100000  LowerLimit=0
  Saturation2 : Saturate  UpperLimit=100000  LowerLimit=0
  Selector : Selector  InputPortWidth=8  IndexOptions=Index vector (dialog)  Indices=[1]  OutputSizes=1
  Sum : Sum  Inputs=++|
  Sum1 : Sum  Inputs=|++
  Sum2 : Sum  Inputs=|++
  Sum3 : Sum  Inputs=|++
  Terminator{,1..2,4} (4 alike) : Terminator  Commented=on
  Terminator{3,5..7} (4 alike) : Terminator
  Three-axis Inertial Measurement Unit3 : aerolibnav/Three-axis Inertial Measurement Unit  units=Metric (MKS)  imu=[0 0 0]  i_Ts=0  dtype_a=on  w_a=190  z_a=0.707  a_sf_cc=[1 0 0; 0 1 0; 0 0 1]  a_bias=[0 0 0]  a_sat="[-160  -160  -160 160 160 160]"  dtype_g=on  w_g=190  z_g=0.707  g_sf_cc=[1 0 0; 0 1 0; 0 0 1]  g_bias=[0 0 0]  g_sens=[0 0 0]  g_sat="[-4.36  -4.36  -4.36 4.36 4.36 4.36]"  i_rand=off  i_seeds=[23093 23094 23095 23096 23097 23098]  i_pow=ModelParam_noisePowerIMU*[0.0000005 0.0000005 0.0000005 0.000000002 0.000000002 0.000000002]
  Transfer Fcn : TransferFcn  Commented=on  Denominator=[0.05 1]
  Uniform Random Number : UniformRandomNumber  Minimum=-2  Maximum=2  Seed=15634  SampleTime=ModelParam_timeSampBaro
  Uniform Random Number1 : UniformRandomNumber  Minimum=-[0.1,0.1,0.2]  Maximum=[0.1,0.1,0.2]  Seed=[12233,645554,678766]  SampleTime=0.004
  Uniform Random Number2 : UniformRandomNumber  Minimum=-[0.01,0.01,0.01]  Maximum=[0.01,0.01,0.01]  Seed=[3243,44556,2334343]  SampleTime=0.004
  Uniform Random Number3 : UniformRandomNumber  Minimum=-[0.01,0.01,0.01]  Maximum=[0.01,0.01,0.01]  Seed=[45465,454534,1234232]  SampleTime=0.004
  Uniform Random Number4 : UniformRandomNumber  Seed=25634  SampleTime=0.01
  World Magnetic Model 2015 : aerolibgravity2/World Magnetic Model  model=WMM2015 V2 (2015-2020)  customFile='WMM2020.COF'  units=Metric (MKS)  time_in=off  month=November  day=3  year=2017  action=Error  h_out=off  dec_out=on  inc_out=off  ti_out=off
      settings: SourceProductBaseCode=AE
  center of gravity : Constant  Value=[0 0 0]
  magDecGain : Gain  Gain=100
  nT2Gauss : Gain  Gain=1E-5
  SensorOut : Outport  VectorParamsAs1DForOutWhenUnconnected=off
  MagDeclination : Outport  Port=2  VectorParamsAs1DForOutWhenUnconnected=off
  acc : Outport  Port=3  VectorParamsAs1DForOutWhenUnconnected=off
  wires:
  center of gravity/1 -> Three-axis Inertial Measurement Unit3/4
  Sum1/1 -> Data Type Conversion2/1
  Sum2/1 -> Data Type Conversion3/1
  Sum3/1 -> Data Type Conversion4/1
  Matrix Multiply2/1 -> Gain_Mag/1
  magDecGain/1 -> Data Type Conversion1/1
  GyroNoiseSwitch3/1(Out1) -> Add2/3
  Product/1 -> Add2/1
  ModelParam.noiseBaroCoupleWithSpeed/1 -> Product/2
  rho/1 -> Dynamic Pressure/2
  windB/1 -> Dynamic Pressure/1
  Uniform Random Number/1 -> Gain5/1
  dwt/1 -> Three-axis Inertial Measurement Unit3/3
  Gain_Mag/1 -> nT2Gauss/1
  Dynamic Pressure/1 -> Gain1/1, Product/1
  pressure/1 -> Terminator3/1
  Add2/1 -> Mux/3, Saturation2/1
  Demux2/3 -> Saturation1/1, Add2/2
  Demux2/2 -> World Magnetic Model 2015/3
  Demux2/1 -> World Magnetic Model 2015/2
  Matrix Multiply1/1 -> Three-axis Inertial Measurement Unit3/5
  DCMbe/1 -> Matrix Multiply2/1, Matrix Multiply1/1
  Gravity/1 -> Matrix Multiply1/2
  Sum/1 -> Mux/2
  Gain/1 -> Mux/1
  Data Type Conversion6/1 -> Bus Creator/15  "fields_updated"
  Constant/1 -> Data Type Conversion6/1
  time_usec/1 -> Bus Creator/1  "time_usec"
  GPSPos/1 -> Demux2/1
  Demux7/2 -> Bus Creator/12  "diff_pressure"
  Demux7/3 -> Bus Creator/13  "pressure_alt"
  Demux6/2 -> Bus Creator/9  "ymag"
  Demux6/3 -> Bus Creator/10  "zmag"
  TempC/1 -> Mux/4
  Mux/1 -> Data Type Conversion5/1
  Demux7/1 -> Bus Creator/11, Display/1  "abs_pressure"
  Demux5/2 -> Bus Creator/6  "ygyro"
  Demux6/1 -> Bus Creator/8  "xmag"
  Demux5/3 -> Bus Creator/7  "zgyro"
  Demux7/4 -> Bus Creator/14  "temperature"
  Demux3/1 -> Bus Creator/2  "xacc"
  Demux3/2 -> Bus Creator/3  "yacc"
  Demux5/1 -> Bus Creator/5  "xgyro"
  Demux3/3 -> Bus Creator/4  "zacc"
  PWMin/1 -> Selector/1
  Ab/1 -> Three-axis Inertial Measurement Unit3/1
  wb/1 -> Three-axis Inertial Measurement Unit3/2
  MotorNoiseScaleCoe/1(NoiseScaleCoe) -> Terminator/1
  Selector/1 -> AccelNoiseGainFunction/1(theta), MagNoiseGainFunction/1(theta), GyroNoiseGainFunction/1(theta)
  AccelNoiseGainFunction/1(Gain) -> Terminator5/1
  Mag Noise/1 -> Gain2/1
  nT2Gauss/1 -> Sum3/1
  Gain8/1 -> GyroNoiseSwitch2/1(In1)
  GyroNoiseSwitch1/1(Out1) -> Sum2/2
  GyroNoiseSwitch2/1(Out1) -> Sum3/2
  Data Type Conversion2/1 -> Demux3/1
  Data Type Conversion3/1 -> Demux5/1
  Data Type Conversion4/1 -> Demux6/1
  Data Type Conversion5/1 -> Demux7/1
  Bus Creator/1 -> SensorOut/1
  Data Type Conversion1/1 -> MagDeclination/1
  Three-axis Inertial Measurement Unit3/1 -> acc/1, Sum1/1
  Three-axis Inertial Measurement Unit3/2 -> Sum2/1
  ISA Atmosphere Model/2 -> Terminator2/1
  ISA Atmosphere Model/4 -> Terminator4/1
  ISA Atmosphere Model/1 -> Terminator1/1
  Gain5/1 -> GyroNoiseSwitch3/1(In1)
  Accel Noise/1 -> Gain3/1
  GyroNoiseSwitch0/1(Out1) -> Sum1/2
  Gyro Noise/1 -> Gain4/1
  GyroNoiseGainFunction/1(Gain) -> Terminator6/1
  MagNoiseGainFunction/1(Gain) -> Terminator7/1
  Uniform Random Number1/1 -> Gain6/1
  Gain7/1 -> GyroNoiseSwitch1/1(In1)
  Uniform Random Number2/1 -> Gain7/1
  Uniform Random Number3/1 -> Gain8/1
  ISA Atmosphere Model/3 -> Gain/1
  Gain6/1 -> GyroNoiseSwitch0/1(In1)
  LowPassFilter2/1(accelDataOut) -> LowPassFilter/1(gyroDataIn)
  Gain9/1 -> GyroNoiseSwitch4/1(In1)
  Uniform Random Number4/1 -> Gain9/1
  Gain1/1 -> Sum/2
  GyroNoiseSwitch4/1(Out1) -> Sum/1
  Saturation1/1 -> World Magnetic Model 2015/1
  Saturation2/1 -> ISA Atmosphere Model/1
  World Magnetic Model 2015/1 -> Matrix Multiply2/2
  World Magnetic Model 2015/2 -> magDecGain/1

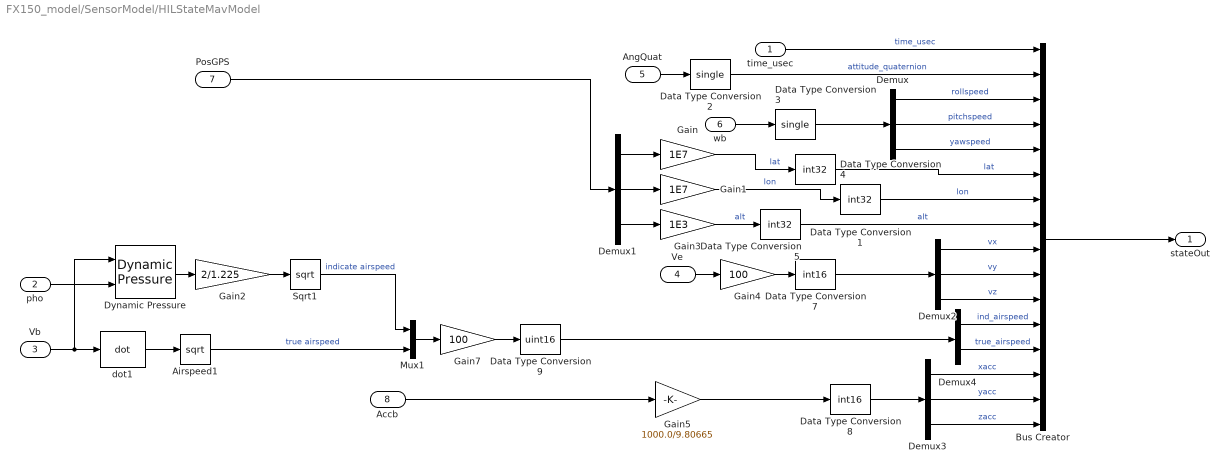
== system FX150_model/SensorModel/HILStateMavModel ==
  time_usec : Inport
  pho : Inport  Port=2
  Vb : Inport  Port=3
  Ve : Inport  Port=4
  AngQuat : Inport  Port=5
  wb : Inport  Port=6
  PosGPS : Inport  Port=7
  Accb : Inport  Port=8
  Airspeed1 : Sqrt  AlgorithmType=Newton-Raphson
  Bus Creator : BusCreator  Inputs=16  OutDataTypeStr=Bus: MavLinkStateQuat  NonVirtualBus=on
  Data Type Conversion1 : DataTypeConversion  OutDataTypeStr=int32  RndMeth=Round  SaturateOnIntegerOverflow=off
  Data Type Conversion2 : DataTypeConversion  OutDataTypeStr=single  SaturateOnIntegerOverflow=off  RndMeth=Floor
  Data Type Conversion3 : DataTypeConversion  OutDataTypeStr=single  SaturateOnIntegerOverflow=off  RndMeth=Floor
  Data Type Conversion4 : DataTypeConversion  OutDataTypeStr=int32  RndMeth=Round  SaturateOnIntegerOverflow=off
  Data Type Conversion5 : DataTypeConversion  OutDataTypeStr=int32  RndMeth=Round  SaturateOnIntegerOverflow=off
  Data Type Conversion7 : DataTypeConversion  OutDataTypeStr=int16  RndMeth=Round  SaturateOnIntegerOverflow=off
  Data Type Conversion8 : DataTypeConversion  OutDataTypeStr=int16  RndMeth=Round  SaturateOnIntegerOverflow=off
  Data Type Conversion9 : DataTypeConversion  OutDataTypeStr=uint16  RndMeth=Round  SaturateOnIntegerOverflow=off
  Demux{,1..3} (4 alike) : Demux  Outputs=3
  Demux4 : Demux  Outputs=2
  Dynamic Pressure : aerolibasang/Dynamic Pressure
  Gain : Gain  Gain=1E7
  Gain1 : Gain  Gain=1E7
  Gain2 : Gain  Gain=2/1.225
  Gain3 : Gain  Gain=1E3
  Gain4 : Gain  Gain=100
  Gain5 : Gain  Gain=1000.0/9.80665
  Gain7 : Gain  Gain=100
  Mux1 : Mux  Inputs=2
  Sqrt1 : Sqrt
  dot1 : aerolibasang/Incidence, Sideslip, & Airspeed/dot  SystemSampleTime=-1  VariantActivationTime=update diagram  Latency=0  AutoFrameSizeCalculation=off
      settings: SourceProductBaseCode=AE
  stateOut : Outport  VectorParamsAs1DForOutWhenUnconnected=off
  wires:
  Sqrt1/1 -> Mux1/1  "indicate airspeed"
  Gain2/1 -> Sqrt1/1
  Dynamic Pressure/1 -> Gain2/1
  time_usec/1 -> Bus Creator/1  "time_usec"
  Vb/1 -> dot1/1, Dynamic Pressure/1
  AngQuat/1 -> Data Type Conversion2/1
  Ve/1 -> Gain4/1
  wb/1 -> Data Type Conversion3/1
  Airspeed1/1 -> Mux1/2  "true airspeed"
  Mux1/1 -> Gain7/1
  Demux4/1 -> Bus Creator/12  "ind_airspeed"
  Demux4/2 -> Bus Creator/13  "true_airspeed"
  Demux3/3 -> Bus Creator/16  "zacc"
  Demux3/2 -> Bus Creator/15  "yacc"
  Demux3/1 -> Bus Creator/14  "xacc"
  Gain5/1 -> Data Type Conversion8/1
  Accb/1 -> Gain5/1
  Demux2/3 -> Bus Creator/11  "vz"
  Demux2/2 -> Bus Creator/10  "vy"
  Demux2/1 -> Bus Creator/9  "vx"
  Gain4/1 -> Data Type Conversion7/1
  Gain3/1 -> Data Type Conversion5/1  "alt"
  Gain1/1 -> Data Type Conversion1/1  "lon"
  Gain/1 -> Data Type Conversion4/1  "lat"
  Demux1/3 -> Gain3/1
  Demux1/2 -> Gain1/1
  Demux1/1 -> Gain/1
  Demux/3 -> Bus Creator/5  "yawspeed"
  Demux/2 -> Bus Creator/4  "pitchspeed"
  Demux/1 -> Bus Creator/3  "rollspeed"
  Data Type Conversion2/1 -> Bus Creator/2  "attitude_quaternion"
  pho/1 -> Dynamic Pressure/2
  Gain7/1 -> Data Type Conversion9/1
  dot1/1 -> Airspeed1/1
  Data Type Conversion3/1 -> Demux/1
  Data Type Conversion7/1 -> Demux2/1
  Data Type Conversion9/1 -> Demux4/1
  Data Type Conversion8/1 -> Demux3/1
  Data Type Conversion4/1 -> Bus Creator/6  "lat"
  Data Type Conversion1/1 -> Bus Creator/7  "lon"
  Data Type Conversion5/1 -> Bus Creator/8  "alt"
  Bus Creator/1 -> stateOut/1
  PosGPS/1 -> Demux1/1

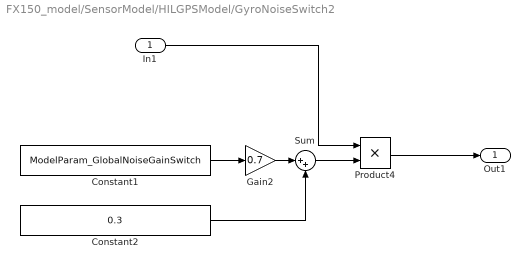
== system FX150_model/SensorModel/HILGPSModel/GyroNoiseSwitch2 ==
  In1 : Inport
  Constant1 : Constant  Value=ModelParam_GlobalNoiseGainSwitch
  Constant2 : Constant  Value=0.3
  Gain2 : Gain  Gain=0.7
  Product4 : Product
  Sum : Sum  Inputs=|++
  Out1 : Outport  VectorParamsAs1DForOutWhenUnconnected=off
  wires:
  Sum/1 -> Product4/2
  Product4/1 -> Out1/1
  Gain2/1 -> Sum/1
  In1/1 -> Product4/1
  Constant1/1 -> Gain2/1
  Constant2/1 -> Sum/2

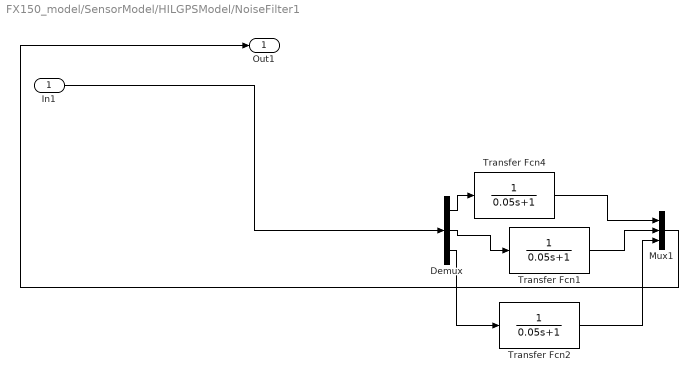
== system FX150_model/SensorModel/HILGPSModel/NoiseFilter1 ==
  In1 : Inport
  Demux : Demux  Outputs=3
  Mux1 : Mux  Inputs=3
  Transfer Fcn1 : TransferFcn  Denominator=[0.05 1]
  Transfer Fcn2 : TransferFcn  Denominator=[0.05 1]
  Transfer Fcn4 : TransferFcn  Denominator=[0.05 1]
  Out1 : Outport  VectorParamsAs1DForOutWhenUnconnected=off
  wires:
  Mux1/1 -> Out1/1
  In1/1 -> Demux/1
  Demux/3 -> Transfer Fcn2/1
  Transfer Fcn4/1 -> Mux1/1
  Transfer Fcn2/1 -> Mux1/3
  Demux/1 -> Transfer Fcn4/1
  Transfer Fcn1/1 -> Mux1/2
  Demux/2 -> Transfer Fcn1/1

== system FX150_model/SensorModel/HILGPSModel/NoiseFilter2 ==
  In1 : Inport
  Demux : Demux  Outputs=3
  Mux1 : Mux  Inputs=3
  Transfer Fcn1 : TransferFcn  Denominator=[0.05 1]
  Transfer Fcn2 : TransferFcn  Denominator=[0.05 1]
  Transfer Fcn4 : TransferFcn  Denominator=[0.05 1]
  Out1 : Outport  VectorParamsAs1DForOutWhenUnconnected=off
  wires:
  Mux1/1 -> Out1/1
  In1/1 -> Demux/1
  Demux/3 -> Transfer Fcn2/1
  Transfer Fcn4/1 -> Mux1/1
  Transfer Fcn2/1 -> Mux1/3
  Demux/1 -> Transfer Fcn4/1
  Transfer Fcn1/1 -> Mux1/2
  Demux/2 -> Transfer Fcn1/1

== system FX150_model/SensorModel/HILSensorMavModel1/GyroNoiseSwitch0 ==
  In1 : Inport
  Constant1 : Constant  Value=ModelParam_GlobalNoiseGainSwitch
  Constant2 : Constant  Value=0.2
  Gain2 : Gain  Gain=0.8
  Product4 : Product
  Sum : Sum  Inputs=|++
  Out1 : Outport  VectorParamsAs1DForOutWhenUnconnected=off
  wires:
  Sum/1 -> Product4/2
  Product4/1 -> Out1/1
  Gain2/1 -> Sum/1
  In1/1 -> Product4/1
  Constant1/1 -> Gain2/1
  Constant2/1 -> Sum/2

== system FX150_model/SensorModel/HILSensorMavModel1/GyroNoiseSwitch1 ==
  In1 : Inport
  Constant1 : Constant  Value=ModelParam_GlobalNoiseGainSwitch
  Constant2 : Constant  Value=0.2
  Gain2 : Gain  Gain=0.8
  Product4 : Product
  Sum : Sum  Inputs=|++
  Out1 : Outport  VectorParamsAs1DForOutWhenUnconnected=off
  wires:
  Sum/1 -> Product4/2
  Product4/1 -> Out1/1
  Gain2/1 -> Sum/1
  In1/1 -> Product4/1
  Constant1/1 -> Gain2/1
  Constant2/1 -> Sum/2

== system FX150_model/SensorModel/HILSensorMavModel1/GyroNoiseSwitch2 ==
  In1 : Inport
  Constant1 : Constant  Value=ModelParam_GlobalNoiseGainSwitch
  Constant2 : Constant  Value=0.2
  Gain2 : Gain  Gain=0.8
  Product4 : Product
  Sum : Sum  Inputs=|++
  Out1 : Outport  VectorParamsAs1DForOutWhenUnconnected=off
  wires:
  Sum/1 -> Product4/2
  Product4/1 -> Out1/1
  Gain2/1 -> Sum/1
  In1/1 -> Product4/1
  Constant1/1 -> Gain2/1
  Constant2/1 -> Sum/2
